simulink model "PowerLimiterModelFinal"  (R2024b)
settings: Solver=VariableStepAuto  StartTime=0.0  StopTime=20  RelTol=1e-3

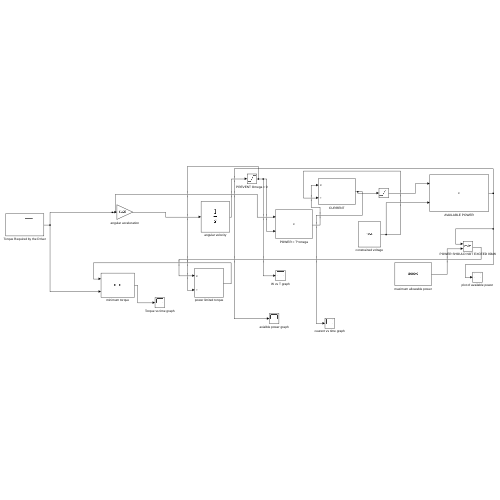
[thumbnail: Simulink's stored preview of the top-level diagram]
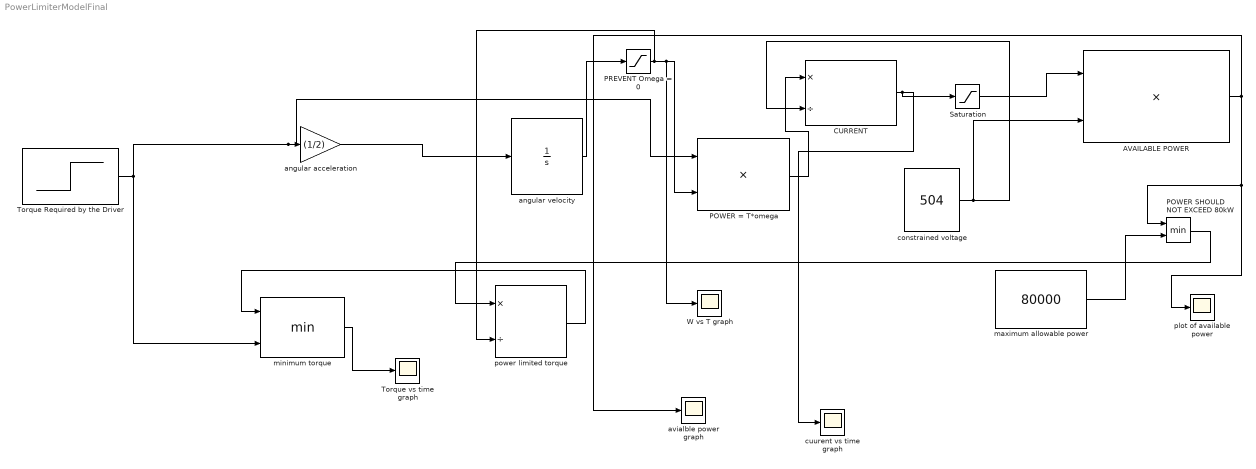
== system PowerLimiterModelFinal ==
  AVAILABLE POWER : Product
  CURRENT : Product  Inputs=*/
  POWER = T*omega : Product
  POWER SHOULD NOT EXCEED 80kW : MinMax  Inputs=2
  PREVENT Omega = 0 : Saturate  UpperLimit=800  LowerLimit=0.1
  Saturation : Saturate  UpperLimit=90  LowerLimit=0
  Torque Required by the Driver : Step  After=100  SampleTime=0
  Torque vs time graph : Scope
  W vs T graph : Scope
  angular acceleration : Gain  Gain=(1/2)
  angular velocity : Integrator
  avialble power graph : Scope
  constrained voltage : Constant  Value=504
  cuurent vs time graph : Scope
  maximum allowable power : Constant  Value=80000
  minimum torque : MinMax  Inputs=2
  plot of available power : Scope
  power limited torque : Product  Inputs=*/
  wires:
  POWER = T*omega/1 -> CURRENT/1
  power limited torque/1 -> minimum torque/1
  minimum torque/1 -> Torque vs time graph/1
  angular velocity/1 -> PREVENT Omega = 0/1
  Torque Required by the Driver/1 -> POWER = T*omega/1, angular acceleration/1, minimum torque/2
  angular acceleration/1 -> angular velocity/1
  PREVENT Omega = 0/1 -> power limited torque/2, W vs T graph/1, POWER = T*omega/2
  constrained voltage/1 -> AVAILABLE POWER/2, CURRENT/2
  CURRENT/1 -> Saturation/1, cuurent vs time graph/1
  AVAILABLE POWER/1 -> avialble power graph/1, plot of available power/1, POWER SHOULD NOT EXCEED 80kW/1
  maximum allowable power/1 -> POWER SHOULD NOT EXCEED 80kW/2
  POWER SHOULD NOT EXCEED 80kW/1 -> power limited torque/1
  Saturation/1 -> AVAILABLE POWER/1
